simulink model "simula_gpc_generic_U"  (R2018a)
settings: Solver=VariableStepAuto  StartTime=0.0  StopTime=Tsim  RelTol=1e-3
values from neighbouring files (symbols this model uses):
  GPC = gpc_tf2ss_U(Pz,[],delta,3,1)    [gpc_generic_U.m]
  Qd = 1*eye(GPC.n*GPC.nout)    [gpc_generic_U.m]
  Ql = lambda*eye(GPC.nu*GPC.nin)    [gpc_generic_U.m]
  Ts = 0.03    [gpc_generic_U.m]
  Tsim = 35    [gpc_generic_U.m]
libraries: simulink x1, cstblocks x1
settings Model: Creator=marcus  LastModifiedBy=marcus

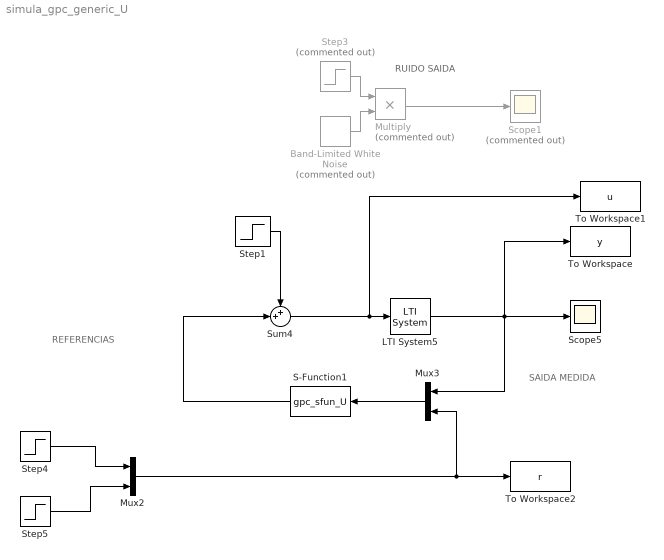
== system simula_gpc_generic_U ==
  note: SAIDA MEDIDA
  note: REFERENCIAS
  note: RUIDO SAIDA
  Band-Limited White Noise : simulink/Sources/Band-Limited White Noise  Commented=on  Cov=Ts/5000  Ts=Ts/10  seed=[23341]
  LTI System5 : cstblocks/LTI System  sys=P  IC=[]
  Multiply : Product  Commented=on
  Mux2 : Mux  Inputs=2
  Mux3 : Mux  Inputs=2
  S-Function1 : S-Function  FunctionName=gpc_sfun_U  Parameters=GPC,Ql,Qd  SFunctionDeploymentMode=off  EnableBusSupport=off
  Scope1 : Scope  Commented=on
  Scope5 : Scope
  Step1 : Step  Time=11  After=-0.1  SampleTime=0
  Step3 : Step  Commented=on  Time=4*Tsim/5  SampleTime=0
  Step4 : Step  Time=0  SampleTime=Ts
  Step5 : Step  Time=Tsim/2  After=0.5  SampleTime=Ts
  Sum4 : Sum  Inputs=++|
  To Workspace : ToWorkspace  VariableName=y  SaveFormat=Timeseries  SampleTime=Ts
  To Workspace1 : ToWorkspace  VariableName=u  SaveFormat=Timeseries  SampleTime=Ts
  To Workspace2 : ToWorkspace  VariableName=r  SaveFormat=Timeseries  SampleTime=-1
  wires:
  Mux2/1 -> Mux3/2, To Workspace2/1
  Mux3/1 -> S-Function1/1
  Sum4/1 -> To Workspace1/1, LTI System5/1
  S-Function1/1 -> Sum4/2
  Step1/1 -> Sum4/1
  Step3/1 -> Multiply/1
  Band-Limited White Noise/1 -> Multiply/2
  LTI System5/1 -> To Workspace/1, Mux3/1, Scope5/1
  Step4/1 -> Mux2/1
  Multiply/1 -> Scope1/1
  Step5/1 -> Mux2/2
